simulink model "Project_6237083_Sharma"  (Simulink 8.0)
settings: Solver=ode45  StartTime=0.0  StopTime=700*Ts  RelTol=1e-3
PreLoadFcn:
  | Ts=20e-9;         % Sample period
  | W = 9;            % Bit-width
  | x_constant = 18;  % Input x
  | gap = 600;        % Gap until signal start goes HIGH again
  | 
  | % Input sequence for x signal
  | x_value = [0 x_constant zeros(1,gap)]';      % value
  | x_time = [0:length(x_value)-1]'*Ts;          % time
  | x = [x_time x_value];                        % signal
  | 
  | % Input sequence for start signal
  | start_value = [0 1 zeros(1,gap)]';           % value
  | start_time = [0:length(start_value)-1]'*Ts;  % time
  | start = [start_time start_value];            % signal
undefined symbols (not defined in the file): xlipgetpartsetting
libraries: xbsIndex_r4 x29
settings Model: Creator=alpha  LastModifiedBy=abs105
settings DataIOCC: SignalLoggingSaveFormat=ModelDataLogs
settings OptimizationCC: InitFltsAndDblsToZero=on
settings DebuggingCC: SaveWithParameterizedLinksMsg=none  SignalResolutionControl=TryResolveAllWithWarning  MultiTaskDSMMsg=warning  MultiTaskCondExecSysMsg=none  FcnCallInpInsideContextMsg=UseLocalSettings  StrictBusMsg=Warning
settings RTWCC: IncludeERTFirstTime=on
settings GRTTargetCC: TargetFcnLib=ansi_tfl_tmw.mat  CombineOutputUpdateFcns=off  GRTInterface=on

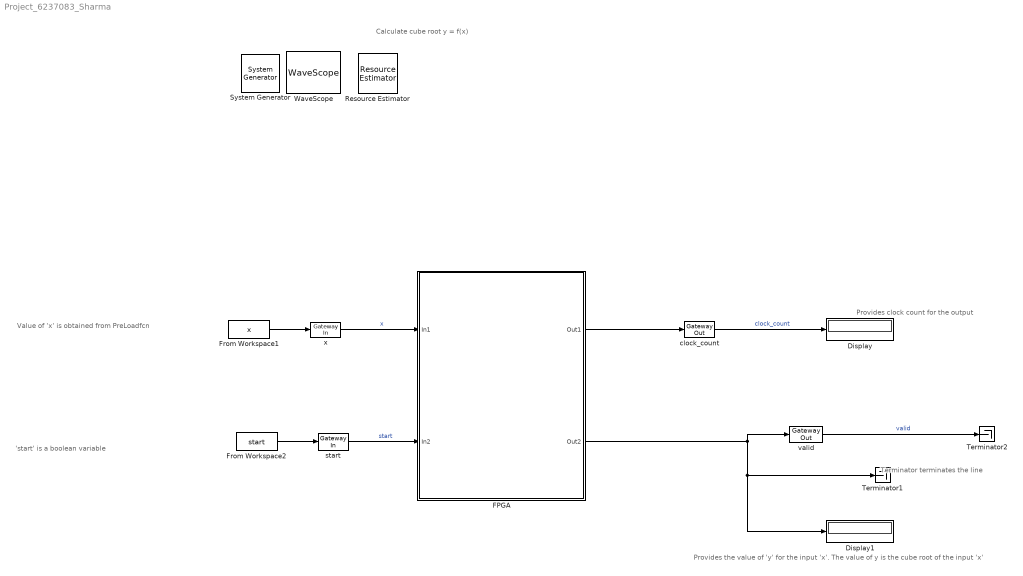
== system Project_6237083_Sharma ==
  note: Terminator terminates the line
  note: Provides the value of 'y' for the input 'x'.
      |                            The value of y is the cube root of the input 'x'
  note: Provides clock count for the output
  note: 'start' is a boolean variable
  note: Value of 'x' is obtained from PreLoadfcn
  note: Calculate cube root y = f(x)
  " System Generator" : xbsIndex_r4/ System Generator  Tag=genX  xilinxfamily=spartan3e  part=xc3s500e  speed=-4  package=fg320  synthesis_tool=XST  clock_wrapper=Clock Enables  directory=./ise  proj_type=Project Navigator  Synth_file=XST Defaults  Impl_file=ISE Defaults  testbench=off  simulink_period=Ts  sysclk_period=20  dcm_input_clock_period=100  incr_netlist=off  trim_vbits=Everywhere in SubSystem  dbl_ovrd=According to Block Masks  core_generation=According to Block Masks  run_coregen=off  deprecated_control=off  eval_field=0  block_type=sysgen
      settings: block_version=8.2.02
  Display : Display
  Display1 : Display
  FPGA : Subsystem
  From Workspace1 : FromWorkspace  VariableName=x  SampleTime=Ts  Interpolate=off  OutputAfterFinalValue=Holding final value
  From Workspace2 : FromWorkspace  VariableName=start  SampleTime=Ts  Interpolate=off  OutputAfterFinalValue=Holding final value
  Resource Estimator : xbsIndex_r4/Resource Estimator  Tag=resEstTag  Slices=0  FFs=0  BRAMs=0  LUTs=0  IOBs=0  EBMs=0  TBUFs=0  xl_use_estimator_area=off  est_options=Estimate  block_type=resource_estimator
      settings: AttributesFormatString=Resource\nEstimator  block_version=11.4
  Terminator1 : Terminator
  Terminator2 : Terminator
  WaveScope : xbsIndex_r4/WaveScope  block_type=wavescope
      settings: block_version=8.2.02
  clock_count : xbsIndex_r4/Gateway Out  inherit_from_input=off  hdl_port=on  timing_constraint=None  locs_specified=off  LOCs={'F9'}  UseAsDAC=off  DACChannel='1'  block_type=gatewayout
      settings: infoedit="Gateway out block.  Converts Xilinx fixed point inputs into ouputs of type Simulink integer, double, or fixed point.<P><P>Hardware notes:  In hardware these blocks become top level output ports or are discarded, depending on how they are configured."  xl_area=[0 0 0 0 16 0 0]  block_version=8.2.02
  start : xbsIndex_r4/Gateway In  gui_display_data_type=Boolean  arith_type=Boolean  n_bits=W  bin_pt=0  preci_type=Single  exp_width=8  frac_width=24  quantization="Round  (unbiased: +/- Inf)"  overflow=Wrap  period=Ts  dbl_ovrd=off  timing_constraint=None  locs_specified=off  LOCs={'V16'}  UseAsADC=off  ADCChannel='1'  inherit_from_input=off  hdl_port=on  block_type=gatewayin
      settings: xl_area=[0 0 0 0 1 0 0]  block_version=8.2.02
  valid : xbsIndex_r4/Gateway Out  inherit_from_input=off  hdl_port=on  timing_constraint=None  locs_specified=off  LOCs={'F9'}  UseAsDAC=off  DACChannel='1'  block_type=gatewayout
      settings: infoedit="Gateway out block.  Converts Xilinx fixed point inputs into ouputs of type Simulink integer, double, or fixed point.<P><P>Hardware notes:  In hardware these blocks become top level output ports or are discarded, depending on how they are configured."  xl_area=[0 0 0 0 1 0 0]  block_version=8.2.02
  x : xbsIndex_r4/Gateway In  gui_display_data_type=Fixed-point  arith_type=Unsigned  n_bits=W  bin_pt=0  preci_type=Single  exp_width=8  frac_width=24  quantization="Round  (unbiased: +/- Inf)"  overflow=Wrap  period=Ts  dbl_ovrd=off  timing_constraint=None  locs_specified=off  LOCs={'V16'}  UseAsADC=off  ADCChannel='1'  inherit_from_input=off  hdl_port=on  block_type=gatewayin
      settings: infoedit="Gateway in block.  Converts inputs of type Simulink integer, double and fixed point to  Xilinx fixed point type.<br><br>Hardware notes:  In hardware these blocks become top level input ports."  xl_area=[0 0 0 0 16 0 0]  block_version=8.2.02
  wires:
  From Workspace1/1 -> x/1
  From Workspace2/1 -> start/1
  FPGA/2(Out2) -> Display1/1, Terminator1/1, valid/1
  valid/1 -> Terminator2/1  "valid"
  clock_count/1 -> Display/1  "clock_count"
  start/1 -> FPGA/2(In2)  "start"
  x/1 -> FPGA/1(In1)  "x"
  FPGA/1(Out1) -> clock_count/1

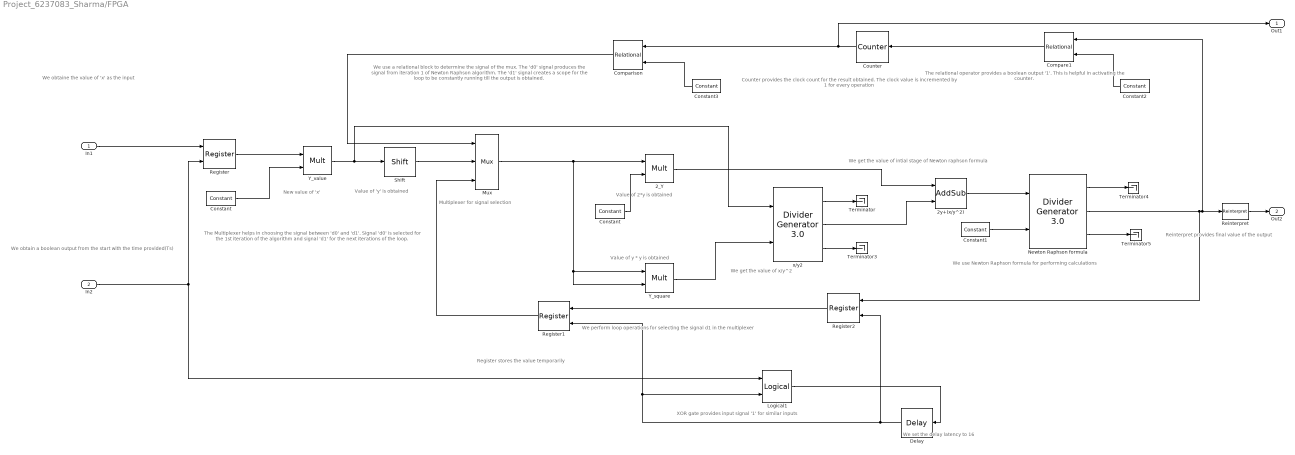
== system Project_6237083_Sharma/FPGA ==
  note: The Multiplexer helps in choosing the signal between 'd0' and 'd1'.
      | Signal 'd0' is selected for the 1st iteration of the algorithm and
      | signal 'd1' for the next iterations of the loop.
  note: Reinterpret provides final value
      |                     of the output
  note: Register stores the value temporarily
  note: We obtain a boolean output from the start with
      |                              the time provided(Ts)
  note: We obtaine the value of 'x' as the input
  note: We use a relational block to determine the signal of the mux.
      | The 'd0' signal produces the signal from iteration 1 of Newton Raphson algorithm.
      | The 'd1' signal creates a scope for the loop to be constantly running till the output is obtained.
  note: The relational operator provides a boolean output '1'.
      |               This is helpful in activating the counter.
  note: Counter provides the clock count for the result obtained.
      |                                          The clock value is incremented by 1 for every operation
  note: We set the delay latency to 16
  note: XOR gate provides input signal '1' for similar inputs
  note: We perform loop operations for selecting the signal d1 in the multiplexer
  note: We use Newton Raphson formula for performing calculations
  note: We get the value of intial stage of Newton raphson formula
  note: We get the value of x/y^2
  note: Value of y * y is obtained
  note: Value of 2*y is obtained
  note: Multiplexer for signal selection
  note: Value of 'y' is obtained
  note: New value of 'x'
  In1 : Inport
  In2 : Inport  Port=2
  2_Y : xbsIndex_r4/Mult  precision=User Defined  arith_type=Unsigned  n_bits=W+5  bin_pt=0  quantization="Round  (unbiased: +/- Inf)"  overflow=Wrap  en=off  latency=0  dbl_ovrd=off  use_behavioral_HDL=off  opt=Speed  use_embedded=on  optimum_pipeline=off  pipeline=on  use_rpm=on  placement_style=Triangular  block_type=mult
  2y+(x/y^2) : xbsIndex_r4/AddSub  mode=Addition  use_carryin=off  use_carryout=off  en=off  latency=0  precision=User Defined  arith_type=Unsigned  n_bits=W+5  bin_pt=0  quantization=Truncate  overflow=Wrap  dbl_ovrd=off  use_behavioral_HDL=off  hw_selection=Fabric  pipelined=off  block_type=addsub
  Compare1 : xbsIndex_r4/Relational  mode=a>b  en=off  latency=0  dbl_ovrd=off  block_type=relational
  Comparison : xbsIndex_r4/Relational  mode=a>=b  en=off  latency=0  dbl_ovrd=off  block_type=relational
  Constant : xbsIndex_r4/Constant  const=8  gui_display_data_type=Fixed-point  arith_type=Unsigned  n_bits=W+5  bin_pt=0  preci_type=Single  exp_width=8  frac_width=24  explicit_period=off  period=1  equ=P=C  opselect=C  inp2=PCIN>>17  opr=+  inp1=P  carry=CIN  dbl_ovrd=off  block_type=constant
  "Constant " : xbsIndex_r4/Constant  const=2  gui_display_data_type=Fixed-point  arith_type=Unsigned  n_bits=W+5  bin_pt=0  preci_type=Single  exp_width=8  frac_width=24  explicit_period=off  period=1  equ=P=C  opselect=C  inp2=PCIN>>17  opr=+  inp1=P  carry=CIN  dbl_ovrd=off  block_type=constant
  Constant1 : xbsIndex_r4/Constant  const=3  gui_display_data_type=Fixed-point  arith_type=Unsigned  n_bits=W+5  bin_pt=0  preci_type=Single  exp_width=8  frac_width=24  explicit_period=off  period=1  equ=P=C  opselect=C  inp2=PCIN>>17  opr=+  inp1=P  carry=CIN  dbl_ovrd=off  block_type=constant
  Constant2 : xbsIndex_r4/Constant  const=1  gui_display_data_type=Fixed-point  arith_type=Unsigned  n_bits=W+5  bin_pt=0  preci_type=Single  exp_width=8  frac_width=24  explicit_period=off  period=1  equ=P=C  opselect=C  inp2=PCIN>>17  opr=+  inp1=P  carry=CIN  dbl_ovrd=off  block_type=constant
  Constant3 : xbsIndex_r4/Constant  const=1  gui_display_data_type=Fixed-point  arith_type=Unsigned  n_bits=W+5  bin_pt=0  preci_type=Single  exp_width=8  frac_width=24  explicit_period=off  period=1  equ=P=C  opselect=C  inp2=PCIN>>17  opr=+  inp1=P  carry=CIN  dbl_ovrd=off  block_type=constant
  Counter : xbsIndex_r4/Counter  cnt_type=Free Running  cnt_to=Inf  operation=Up  start_count=0  cnt_by_val=1  arith_type=Unsigned  n_bits=W+5  bin_pt=0  load_pin=off  rst=off  en=on  explicit_period=on  period=Ts  dbl_ovrd=off  use_behavioral_HDL=off  implementation=Fabric  block_type=counter
  Delay : xbsIndex_r4/Delay  rst=off  infoeditControl=Selection of Reset will increase slice count due to use of real FFs and instead of SRLs  en=off  latency=16  dbl_ovrd=off  reg_retiming=off  block_type=delay
  Logical1 : xbsIndex_r4/Logical  logical_function=XNOR  inputs=2  en=off  latency=0  precision=Full  arith_type=Unsigned  n_bits=16  bin_pt=0  align_bp=on  dbl_ovrd=off  block_type=logical
  Mux : xbsIndex_r4/Mux  inputs=2  en=off  latency=0  precision=Full  arith_type=Unsigned  n_bits=16  bin_pt=14  quantization=Truncate  overflow=Wrap  dbl_ovrd=off  block_type=mux
  Newton Raphson formula : xbsIndex_r4/Divider Generator 3.0   dividend_and_quotient_width=W+5  divisor_width=W+5  algorithm_type=Radix2  remainder_type=Remainder  fractional_width=19  clocks_per_division=1  divide_by_zero_detect=off  latency_configuration=Automatic  latency=16  ce=off  sclr=off  sclr_ce_priority=SCLR_overrides_CE  operand_sign=Signed  ip_name=Divider Generator  ip_version=3.0  dsptool_ready=true  wrapper_available=true  port_translation_map={ 'ce' => 'en', 'sclr' => 'rst' }  ipcore_fpga_part=xlipgetpartsetting(gcb, {'virtex4', 'xc4vsx35', '-10', 'ff668'})  ipcore_verbose=false  block_type=div_gen_v3_0
  Register : xbsIndex_r4/Register  init=0  rst=off  en=on  dbl_ovrd=off  block_type=register
  Register1 : xbsIndex_r4/Register  init=0  rst=off  en=on  dbl_ovrd=off  block_type=register
  Register2 : xbsIndex_r4/Register  init=0  rst=off  en=on  dbl_ovrd=off  block_type=register
  Reinterpret : xbsIndex_r4/Reinterpret  force_arith_type=off  arith_type=Unsigned  force_bin_pt=on  bin_pt=1  block_type=reinterpret
  Shift : xbsIndex_r4/Shift  shift_dir=Right  shift_bits=1  en=off  latency=0  precision=Full  arith_type="Signed  (2's comp)"  n_bits=16  bin_pt=14  quantization=Truncate  overflow=Wrap  dbl_ovrd=off  block_type=shift
  Terminator{,3..5} (4 alike) : Terminator
  Y_square : xbsIndex_r4/Mult  precision=User Defined  arith_type=Unsigned  n_bits=W+5  bin_pt=0  quantization=Truncate  overflow=Wrap  en=off  latency=0  dbl_ovrd=off  use_behavioral_HDL=off  opt=Speed  use_embedded=on  optimum_pipeline=off  pipeline=on  use_rpm=on  placement_style=Triangular  block_type=mult
  Y_value : xbsIndex_r4/Mult  precision=User Defined  arith_type=Unsigned  n_bits=W+5  bin_pt=0  quantization=Truncate  overflow=Wrap  en=off  latency=0  dbl_ovrd=off  use_behavioral_HDL=off  opt=Speed  use_embedded=on  optimum_pipeline=off  pipeline=on  use_rpm=on  placement_style=Triangular  block_type=mult
  "x/y2 " : xbsIndex_r4/Divider Generator 3.0   dividend_and_quotient_width=W+5  divisor_width=W+5  algorithm_type=Radix2  remainder_type=Remainder  fractional_width=19  clocks_per_division=1  divide_by_zero_detect=off  latency_configuration=Automatic  latency=16  ce=off  sclr=off  sclr_ce_priority=SCLR_overrides_CE  operand_sign=Signed  ip_name=Divider Generator  ip_version=3.0  dsptool_ready=true  wrapper_available=true  port_translation_map={ 'ce' => 'en', 'sclr' => 'rst' }  ipcore_fpga_part=xlipgetpartsetting(gcb, {'virtex4', 'xc4vsx35', '-10', 'ff668'})  ipcore_verbose=false  block_type=div_gen_v3_0
  Out1 : Outport
  Out2 : Outport  Port=2
  wires:
  Logical1/1 -> Delay/1
  Constant2/1 -> Compare1/2
  Compare1/1 -> Counter/1
  Comparison/1 -> Mux/1
  Newton Raphson formula/2 -> Register2/1, Compare1/1, Reinterpret/1
  Reinterpret/1 -> Out2/1
  "x/y2 "/2 -> 2y+(x/y^2)/2
  2_Y/1 -> 2y+(x/y^2)/1
  Y_square/1 -> "x/y2 "/2
  "x/y2 "/3 -> Terminator3/1
  2y+(x/y^2)/1 -> Newton Raphson formula/1
  "x/y2 "/1 -> Terminator/1
  Register1/1 -> Mux/3
  Register/1 -> Y_value/1
  Constant/1 -> Y_value/2
  Constant3/1 -> Comparison/2
  Mux/1 -> Y_square/2, Y_square/1, 2_Y/1
  "Constant "/1 -> 2_Y/2
  Counter/1 -> Out1/1, Comparison/1
  Shift/1 -> Mux/2
  Y_value/1 -> "x/y2 "/1, Shift/1
  In2/1 -> Register/2, Logical1/1
  In1/1 -> Register/1
  Delay/1 -> Register2/2, Register1/2, Logical1/2
  Constant1/1 -> Newton Raphson formula/2
  Newton Raphson formula/3 -> Terminator5/1
  Register2/1 -> Register1/1
  Newton Raphson formula/1 -> Terminator4/1
